simulink model "Week10_Discussion_Inclass"  (R2022b)
settings: Solver=VariableStepAuto  StartTime=0.0  StopTime=10.0  RelTol=1e-3
undefined symbols (not defined in the file or in its folder): getM, K_d, K_p, q_d, q_i
settings Model: Creator=39638  LastModifiedBy=39638

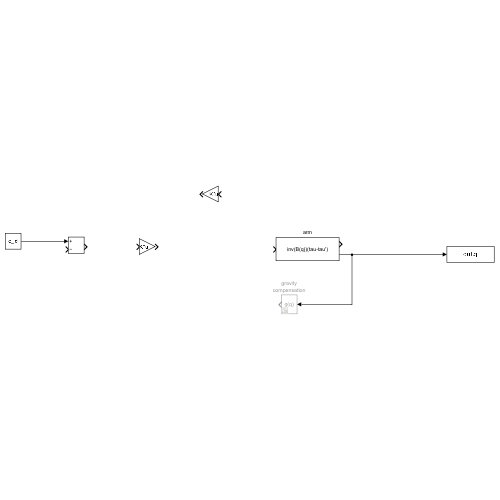
[thumbnail: Simulink's stored preview of the top-level diagram]
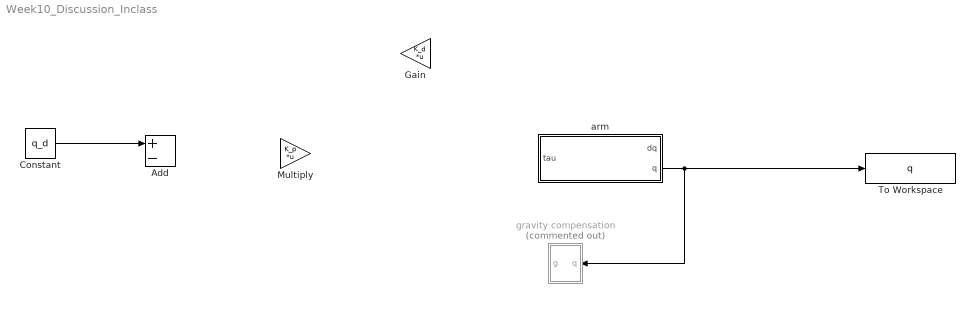
== system Week10_Discussion_Inclass ==
  Add : Sum  Inputs=+-
  Constant : Constant  Value=q_d
  Gain : Gain  Gain=K_d  Multiplication=Matrix(K*u)
  Multiply : Gain  Gain=K_p  Multiplication=Matrix(K*u)
  To Workspace : ToWorkspace  VariableName=q  SaveFormat=Timeseries  SampleTime=-1
  arm : Subsystem
      mask Display: disp('inv(B(q))(tau-tau'')')
  gravity compensation : Subsystem  Commented=on
      mask Display: disp('g(q)')
  wires:
  arm/2("q ") -> To Workspace/1, gravity compensation/1(q)
  Constant/1 -> Add/1

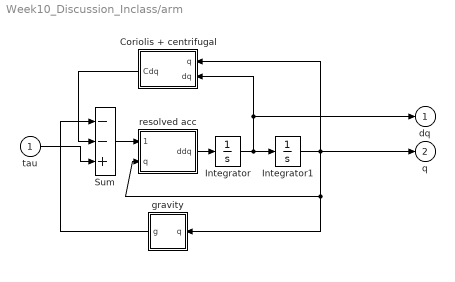
== system Week10_Discussion_Inclass/arm ==
  tau : Inport
  Coriolis + centrifugal : Subsystem
      mask Display: disp('C(q,dq)dq')
  Integrator : Integrator  InitialCondition=[0 0]  ZeroCross=off
  Integrator1 : Integrator  InitialCondition=q_i  ZeroCross=off
  Sum : Sum  Inputs=--+  InputSameDT=on  SaturateOnIntegerOverflow=on  OutDataTypeStr=Inherit: Same as first input
  gravity : Subsystem
      mask Display: disp('g(q)')
  resolved acc : Subsystem
      mask Display: disp('inv(B(q))')
  dq : Outport  InitialOutput=0
  "q " : Outport  Port=2  InitialOutput=0
  wires:
  Coriolis + centrifugal/1(Cdq) -> Sum/2
  tau/1 -> Sum/3
  Integrator1/1 -> Coriolis + centrifugal/1(q), resolved acc/2(q), gravity/1(q), "q "/1
  resolved acc/1(ddq) -> Integrator/1
  Integrator/1 -> Integrator1/1, Coriolis + centrifugal/2(dq), dq/1
  Sum/1 -> resolved acc/1(tau-tau')
  gravity/1(g) -> Sum/1

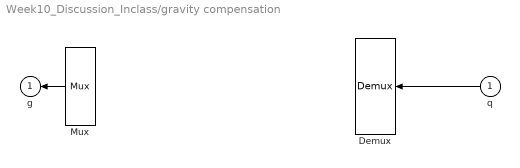
== system Week10_Discussion_Inclass/gravity compensation ==
  q : Inport
  Demux : Demux  Outputs=2
      settings: DisplayOption=none
  Mux : Mux  Inputs=2
  g : Outport  InitialOutput=0
  wires:
  Mux/1 -> g/1
  q/1 -> Demux/1

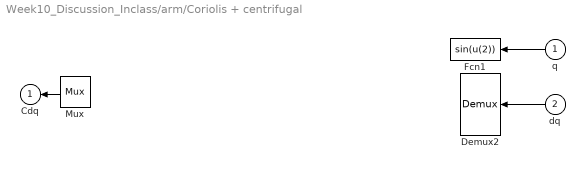
== system Week10_Discussion_Inclass/arm/Coriolis + centrifugal ==
  q : Inport
  dq : Inport  Port=2
  Demux2 : Demux  Outputs=2
      settings: DisplayOption=none
  Fcn1 : Fcn  Expr=sin(u(2))
  Mux : Mux  Inputs=2
  Cdq : Outport  InitialOutput=0
  wires:
  dq/1 -> Demux2/1
  Mux/1 -> Cdq/1
  q/1 -> Fcn1/1

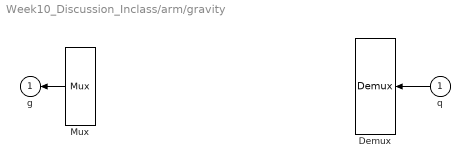
== system Week10_Discussion_Inclass/arm/gravity ==
  q : Inport
  Demux : Demux  Outputs=2
      settings: DisplayOption=none
  Mux : Mux  Inputs=2
  g : Outport  InitialOutput=0
  wires:
  q/1 -> Demux/1
  Mux/1 -> g/1

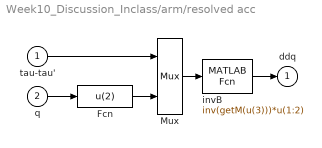
== system Week10_Discussion_Inclass/arm/resolved acc ==
  tau-tau' : Inport
  q : Inport  Port=2
  Fcn : Fcn  Expr=u(2)
  Mux : Mux  Inputs=[2,1]
  "invB " : MATLABFcn  MATLABFcn=inv(getM(u(3)))*u(1:2)  OutputDimensions=2
      mask Display: disp('inv(B(q))')
  ddq : Outport  InitialOutput=0
  wires:
  q/1 -> Fcn/1
  "invB "/1 -> ddq/1
  tau-tau'/1 -> Mux/1
  Mux/1 -> "invB "/1
  Fcn/1 -> Mux/2
